simulink library "uavsimBlockset_UAV3DInterface"  (Simulink 8.6)
settings: Solver=ode45  StartTime=0.0  StopTime=10.0  RelTol=1e-3
libraries: dspnetwork x1
settings Model: Creator=mstolle  LastModifiedBy=j.bolting

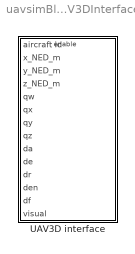
== system uavsimBlockset_UAV3DInterface ==
  UAV3D interface : Subsystem  mask{ip='localhost', udpport=4445}
      mask prompts: ip "IP address"; udpport "UDP port"
      mask init:
      | ip = 'localhost';

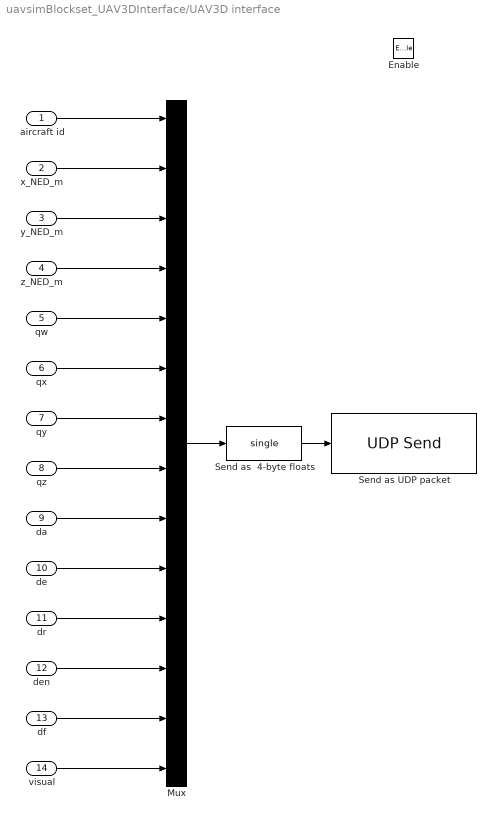
== system uavsimBlockset_UAV3DInterface/UAV3D interface ==
  aircraft id : Inport
  x_NED_m : Inport  Port=2
  y_NED_m : Inport  Port=3
  z_NED_m : Inport  Port=4
  qw : Inport  Port=5
  qx : Inport  Port=6
  qy : Inport  Port=7
  qz : Inport  Port=8
  da : Inport  Port=9
  de : Inport  Port=10
  dr : Inport  Port=11
  den : Inport  Port=12
  df : Inport  Port=13
  visual : Inport  Port=14
  Enable : EnablePort  StatesWhenEnabling=reset
  Mux : Mux  Inputs=14
  Send as  4-byte floats : DataTypeConversion  OutDataTypeStr=single  SaturateOnIntegerOverflow=on  LockScale=on
  Send as UDP packet : dspnetwork/UDP Send  remoteURL=ip  remotePort=udpport  localURL='0.0.0.0'  localPortSource=Automatically determine  localPort=-1  sampletime=-1  separateLengthPort=0
  wires:
  visual/1 -> Mux/14
  Send as  4-byte floats/1 -> Send as UDP packet/1
  Mux/1 -> Send as  4-byte floats/1
  aircraft id/1 -> Mux/1
  y_NED_m/1 -> Mux/3
  qw/1 -> Mux/5
  qy/1 -> Mux/7
  z_NED_m/1 -> Mux/4
  qx/1 -> Mux/6
  x_NED_m/1 -> Mux/2
  qz/1 -> Mux/8
  de/1 -> Mux/10
  da/1 -> Mux/9
  dr/1 -> Mux/11
  den/1 -> Mux/12
  df/1 -> Mux/13
